simulink model "pcssp_varPID"  (R2021b)
settings: configuration reference "configurationSettings" (kept outside this file)
model workspace (MAT data in the model file):
  tp = Simulink.Parameter
  tp.Value.enable = 1
  tp.Value.P = [50 0 0]
  tp.Value.I = [3 0 0]
  tp.Value.D = [0 0 0]
  tp.DataType = 'struct'
  tp.Complexity = 'real'
  tp.Dimensions = [1 1]
undefined symbols (not defined in the file or in its folder): pcssp_varPID_fp, pcssp_varPID_tp
libraries: slpidlib x1
settings Model: DataDictionary=pcssp_varPID.sldd  ParameterArgumentNames=tp  Creator=ravenst1  LastModifiedBy=ravenst1
settings ConfigSetRef: SourceName=configurationSettings

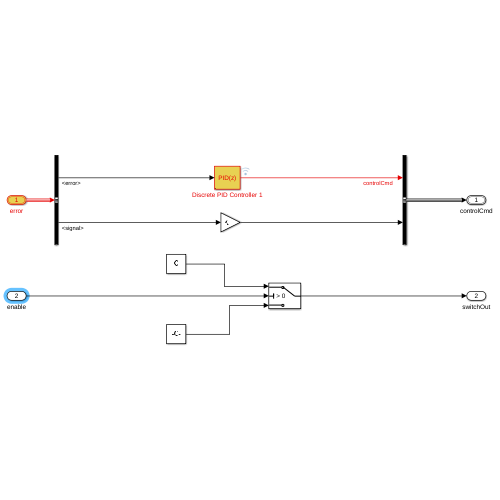
[thumbnail: Simulink's stored preview of the top-level diagram]
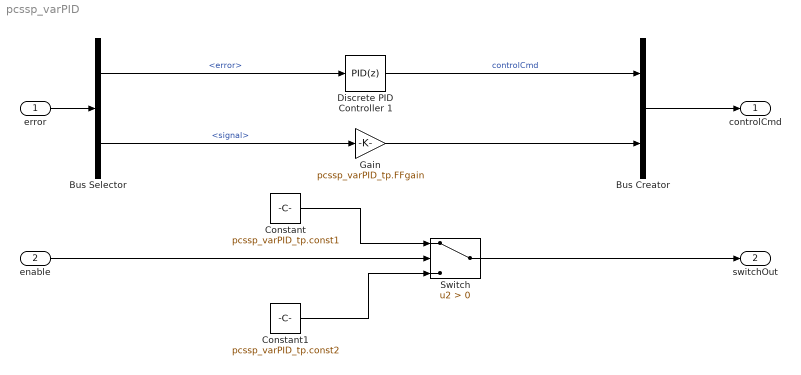
== system pcssp_varPID ==
  error : Inport  OutDataTypeStr=Bus: pcssp_varPID_inBus  SampleTime=pcssp_varPID_fp.timing.dt  Interpolate=off
  enable : Inport  Port=2  OutDataTypeStr=boolean
  Bus Creator : BusCreator  Inputs=2  OutDataTypeStr=Bus: pcssp_varPID_outBus
      settings: InheritFromInputs=off
  Bus Selector : BusSelector  OutputSignals=error,signal
  Constant : Constant  Value=pcssp_varPID_tp.const1
  Constant1 : Constant  Value=pcssp_varPID_tp.const2
  Discrete PID Controller 1 : slpidlib/PID Controller  Controller=PID  Form=Parallel  TimeDomain=Discrete-time  UseExternalTs=off  SampleTime=-1  IntegratorMethod=Forward Euler  FilterMethod=Forward Euler  ControllerParametersSource=internal  P=pcssp_varPID_tp.P  I=pcssp_varPID_tp.I  D=pcssp_varPID_tp.D  UseFilter=on  N=100  TunerSelectOption=Transfer Function Based (PID Tuner App)  InitialConditionSource=internal  InitialConditionForIntegrator=0  InitialConditionForFilter=0  DifferentiatorICPrevScaledInput=0  ExternalReset=none  TrackingMode=off  Kt=1  LimitOutput=off  SatLimitsSource=internal  UpperSaturationLimit=inf  LowerSaturationLimit=-inf  LinearizeAsGain=off  AntiWindupMode=none  Kb=1  POutMin=[]  POutMax=[]  IOutMin=[]  IOutMax=[]  DOutMin=[]  DOutMax=[]  NOutMin=[]  NOutMax=[]  SumOutMin=[]  SumOutMax=[]  SaturationOutMin=[]  SaturationOutMax=[]  PParamMin=[]  PParamMax=[]  IParamMin=[]  IParamMax=[]  DParamMin=[]  DParamMax=[]  NParamMin=[]  NParamMax=[]  KbParamMin=[]  KbParamMax=[]  KtParamMin=[]  KtParamMax=[]  KbOutMin=[]  KbOutMax=[]  KtOutMin=[]  KtOutMax=[]  IntegratorOutMin=[]  IntegratorOutMax=[]  FilterOutMin=[]  FilterOutMax=[]  SumI1OutMin=[]  SumI1OutMax=[]  SumI2OutMin=[]  SumI2OutMax=[]  SumI3OutMin=[]  SumI3OutMax=[]  SumI4OutMin=[]  SumI4OutMax=[]  SumDOutMin=[]  SumDOutMax=[]  DifferentiatorOutMin=[]  DifferentiatorOutMax=[]  FilterDiffOutCoefMin=[]  FilterDiffOutCoefMax=[]  ReciprocalOutMin=[]  ReciprocalOutMax=[]  SumDenOutMin=[]  SumDenOutMax=[]  SumNumOutMin=[]  SumNumOutMax=[]  DivideOutMin=[]  DivideOutMax=[]  UdiffTsProdOutMin=[]  UdiffTsProdOutMax=[]  NTsProdOutMin=[]  NTsProdOutMax=[]  UintegralTsProdOutMin=[]  UintegralTsProdOutMax=[]  UngainTsProdOutMin=[]  UngainTsProdOutMax=[]  IntegratorContinuousStateAttributes=''  IntegratorStateMustResolveToSignalObject=off  IntegratorRTWStateStorageClass=Auto  FilterContinuousStateAttributes=''  FilterStateMustResolveToSignalObject=off  FilterRTWStateStorageClass=Auto  ParallelPVariant=InternalParameters  IdealPVariant=Disabled  IVariant=InternalParameters  DVariant=InternalParameters  IntegratorVariant=Discrete  SatVariant=Disabled  AWVariant=Passthrough  PCopyVariant=Disabled  TRVariant=Disabled  FdbkBlocksVariant=Forward  IdealPFdbkVariant=Disabled  SatFdbkVariant=Disabled  DerivativeFilterVariant=ForwardEulerFilter  NVariant=InternalParameters  NCopyVariant=Disabled  FilterICVariant=InternalICsFilter  IntegratorICVariant=InternalICs  ExternalResetVariant=Disabled  TRSumVariant=Passthrough  SumFdbkVariant=Disabled  SumVariant=Sum_PID  TsampFilterVariant=InternalTs  TsampNgainVariant=Passthrough  TsampIntegralVariant=Passthrough  ExternalSaturationOutDataTypeStr=Inherit: Same as second input
  Gain : Gain  Gain=pcssp_varPID_tp.FFgain
  Switch : Switch  Criteria=u2 > Threshold
  controlCmd : Outport  OutDataTypeStr=Bus: pcssp_varPID_outBus
  switchOut : Outport  Port=2
  wires:
  error/1 -> Bus Selector/1
  Bus Creator/1 -> controlCmd/1
  Bus Selector/1 -> Discrete PID Controller 1/1  "<error>"
  Discrete PID Controller 1/1 -> Bus Creator/1  "controlCmd"
  Bus Selector/2 -> Gain/1  "<signal>"
  Gain/1 -> Bus Creator/2
  enable/1 -> Switch/2
  Constant1/1 -> Switch/3
  Constant/1 -> Switch/1
  Switch/1 -> switchOut/1
